simulink model "MSDRPrimaryLoop_LoadFollow"  (R2021b)
settings: Solver=VariableStepAuto  StartTime=0.0  StopTime=604900  MaxStep=1  MinStep=0.01  RelTol=1e-3
undefined symbols (not defined in the file): a_f, A_free_PHX, a_g, A_h_PHX, beta, beta_t, bubbleGeneratorArea, bubbleGeneratorDh, bubbleGeneratorElevation, bubbleGeneratorLength, bubbleGeneratorVolume, bubbleSaturationLevel, bubbleSeparatorArea, bubbleSeparatorDiameter, bubbleSeparatorDo, bubbleSeparatorLength, bubbleSeparatorSlope, bypassRatio, C0, coreFlowArea, coreFuelVolume, coreLowerPlenumArea, coreLowerPlenumHydraulicDiameter, coreLowerPlenumLength, coreLowerPlenumVolume, coreUpperPlenumArea, coreUpperPlenumHydraulicDiameter, coreUpperPlenumLength, coreUpperPlenumVolume, coreVolume, cpGraphite, dissolusionRatio, dMin, dScale, dsmConst, DXeG, Fiss_factor, fuelChannelHydrualicDiameter, fuelChannelLength, fuelDepositRatio, fuelFraction, fuelGraphiteArea, fuelGraphiteHeatTransferCoefficient, gamma0, gamma1, gamma2, generatorDsm, graphiteKDiff, graphiteUnitCellThickness, initialIodineConcentration, InitialXeMolarConcentration, InjectionRatio, injectionRatio, iodineDecayConstant, IodineDecayConstant, iodineYield, kGraphite, kScale, Lam, lam ... (+60)
libraries: fl_lib x268, nesl_utility x106, SimscapeFluids_lib x20, slpidlib x1
(part 1 of 12)
settings Model: PacingRate=4  Creator=silen  LastModifiedBy=silen
settings SolverCC: ZeroCrossAlgorithm=Adaptive
settings DataIOCC: InitialState=xFinal  SaveFinalState=on  SaveOperatingPoint=on  SaveOutput=off  SignalLogging=off  DSMLogging=off  SaveTime=off  ReturnWorkspaceOutputs=off
settings SimscapeCC: SimscapeLogOpenViewer=on

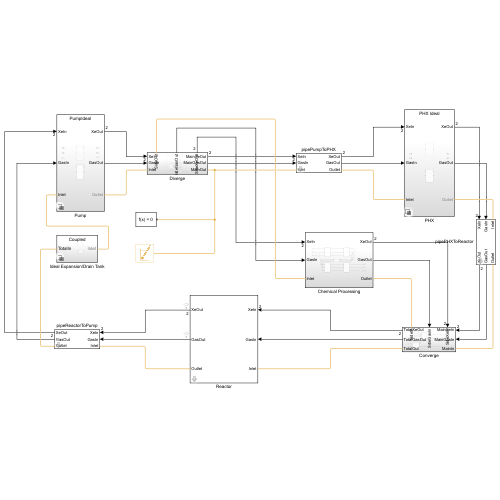
[thumbnail: Simulink's stored preview of the top-level diagram]
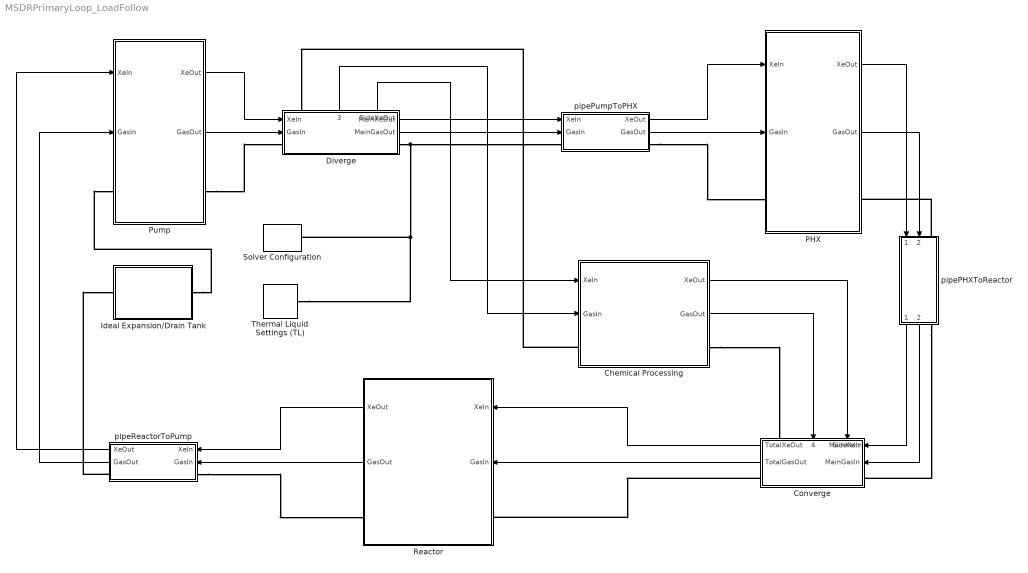
== system MSDRPrimaryLoop_LoadFollow ==
  Chemical Processing : Subsystem
  Converge : Subsystem
      settings: PortSchema="{\"entries\":[{\"content\":{\"sides\":[{\"content\":{\"connectorIds\":[\"In1\",\"In2\",\"LConn1\"]},\"type\":\"ConnectorPlacement.EquallySpacedRectSide\",\"uuid\":\"45a27f6f-7483-4dd0-a911-98512286657b\"},{\"content\":{\"connectorIds\":[\"Out1\",\"Out2\",\"RConn1\"],\"side\":\"RIGHT\"},\"type\":\"ConnectorPlacement.EquallySpacedRectSide\",\"uuid\":\"648a7517-4264-4847-9228-e879d02b25f7\"},{\"content\":{\"connectorIds\":[\"In3\",\"In4\",\"LConn2\"],\"side\":\"TOP\"},\"type\":\"ConnectorPlacement.EquallySpacedRectSide\",\"uuid\":\"a562fb08-ad05-4981-ab1e-7002bfac102c\"},{\"content\":{\"connectorIds\":[],\"side\":\"BOTTOM\"},\"type\":\"ConnectorPlacement.EquallySpacedRectSide\",\"uuid\":\"59ea555a-4c64-4ddd-ae1f-9e1e4b34dfa6\"}]},\"type\":\"ConnectorPlacement.EquallySpacedConnector\",\"uuid\":\"c238e19d-8d7c-41cb-8a15-012ebc62f205\"}],\"packageUris\":[\"http://schema.mathworks.com/mf0/Connector/R2020b\"],\"version\":\"1.0\"}"
  Diverge : Subsystem
      settings: PortSchema="{\"entries\":[{\"content\":{\"sides\":[{\"content\":{\"connectorIds\":[\"In1\",\"In2\",\"LConn1\"]},\"type\":\"ConnectorPlacement.EquallySpacedRectSide\",\"uuid\":\"f25232e3-ff44-4b09-8127-0a17cdec3bda\"},{\"content\":{\"connectorIds\":[\"Out1\",\"Out2\",\"RConn1\"],\"side\":\"RIGHT\"},\"type\":\"ConnectorPlacement.EquallySpacedRectSide\",\"uuid\":\"2b744e7f-4690-47f4-bf66-293fed6e3799\"},{\"content\":{\"connectorIds\":[\"LConn2\",\"Out3\",\"Out4\"],\"side\":\"TOP\"},\"type\":\"ConnectorPlacement.EquallySpacedRectSide\",\"uuid\":\"256231dc-6d03-4995-a517-f1093dd3b2d7\"}]},\"type\":\"ConnectorPlacement.EquallySpacedConnector\",\"uuid\":\"cecb1d8e-0e0f-4899-85a3-e553206939ed\"}],\"packageUris\":[\"http://schema.mathworks.com/mf0/Connector/R2020b\"],\"version\":\"1.0\"}"
  Ideal Expansion/Drain Tank : Subsystem  Variant=on  VariantControlMode=label  VariantControl=Choice  LabelModeActiveChoice=Couple
  PHX : Subsystem  Variant=on  VariantControlMode=label  VariantControl=Choice  LabelModeActiveChoice=Ideal
  Pump : Subsystem  Variant=on  VariantControlMode=label  VariantControl=Choice  LabelModeActiveChoice=Ideal
  Reactor : Subsystem  mask{ReactorPower=thermalPower, NeutronFlux=nominalNeutronFlux}
      mask prompts: ReactorPower "Rated Thermal Power"; NeutronFlux "Nominal Neutron Flux"
  Solver Configuration : nesl_utility/Solver Configuration  PhysicalDomain=network_engine_domain  SubClassName=solver  LeftPortType=input  RightPortType=generic  Tones=[]  Harmonics=[]  SimulateNoise=off  Profile=off  UseLocalSampling=off  EnableSwitchedLinearOptims=on  FrequencyDomain=off  UseCCode=off  RelTol=0.001  AbsTol=1e-06  MinStep=1e-09  ToWorkspace=off  RevertToSquareIcSolve=off  NumHomotopyIterations=100  PhasorMode=off  PhasorModeNumHarmonics=1  DoDC=off  ResidualTolerance=1e-5  UseLocalSolver=on  LocalSolverChoice=NE_BACKWARD_EULER_ADVANCER  LocalSolverSampleTime=1  DoFixedCost=off  MaxNonlinIter=3  MaxModeIter=2  ComputeImpulses=off  ImpulseIterations=2  LinearAlgebra=auto  EquationFormulation=NE_TIME_EF  DelaysMemoryBudget=1024  AutomaticFiltering=on  FilteringTimeConstant=0.001  PartitionStorageMethod=AS_NEEDED  PartitionMemoryBudget=1024  PartitionMethod=ROBUST
      settings: SourceProductBaseCode=PW,SS
  Thermal Liquid Settings (TL) : fl_lib/Thermal Liquid/Utilities/Thermal Liquid Settings (TL)  table_dimensions=foundation.enum.table_dimensions_TL.one_dimensional  T_TLU=temperatureList K  p_TLU=[0.01, 0.1, 5 : 5 : 50] MPa  p_atm=0.1 MPa  pT_region_flag=foundation.enum.pT_region_TL.min_max  T_min=273.16 K  T_max=363.16 K  p_min=0.05 MPa  p_max=50 MPa  T_min_1D=434+273.15 K  T_max_1D=2000+273.15 K  p_min_1D=1 Pa  p_max_1D=10000 MPa  pT_validity_TLU=[1, 1, 1, 1, 1, 1, 1, 1, 1, 1, 1, 1; 1, 1, 1, 1, 1, 1, 1, 1, 1, 1, 1, 1; 1, 1, 1, 1, 1, 1, 1, 1, 1, 1, 1, 1; 1, 1, 1, 1, 1, 1, 1, 1, 1, 1, 1, 1; 1, 1, 1, 1, 1, 1, 1, 1, 1, 1, 1, 1; 0, 1, 1, 1, 1, 1, 1, 1, 1, 1, 1, 1; 0, 1, 1, 1, 1, 1, 1, 1, 1, 1, 1, 1; 0, 1, 1, 1, 1, 1, 1, 1, 1, 1, 1, 1; 0, 1, 1, 1, 1, 1, 1, 1, 1, 1, 1, 1; 0, 1, 1, 1, 1, 1, 1, 1, 1, 1, 1, 1; 0, 0, 1, 1, 1, 1, 1, 1, 1, 1, 1, 1]  rho_parameterization_2D=foundation.enum.rho_parameterization_2D.rho_beta_alpha  rho_parameterization_1D=foundation.enum.rho_parameterization_1D.rho_vector  rho_TLU=[999.7973, 999.8431, 1002.3216, 1004.8218, 1007.293, 1009.7358, 1012.1506, 1014.5379, 1016.8979, 1019.2311, 1021.538, 1023.8188; 999.6579, 999.7009, 1002.0303, 1004.382, 1006.7084, 1009.0101, 1011.2874, 1013.5407, 1015.7703, 1017.9766, 1020.1599, 1022.3206; 998.1632, 998.2045, 1000.4375, 1002.6924, 1004.9239, 1007.1324, 1009.3183, 1011.4819, 1013.6236, 1015.7438, 1017.8428, 1019.921; 995.6057, 995.6458, 997.81864, 1000.0128, 1002.1841, 1004.3332, 1006.4603, 1008.566, 1010.6505, 1012.7144, 1014.758, 1016.7815; 992.1724, 992.2119, 994.35133, 996.5113, 998.6484, 1000.7633, 1002.8563, 1004.928, 1006.9788, 1009.009, 1011.0192, 1013.0097; 988.02, 988.0299, 990.15684, 992.3035, 994.4268, 996.5273, 998.6056, 1000.6622, 1002.6976, 1004.7123, 1006.7067, 1008.6813; 983.18, 983.1901, 985.3217, 987.4721, 989.5983, 991.7008, 993.7803, 995.8374, 997.8726, 999.8864, 1001.8795, 1003.8522; 977.75, 977.7583, 979.9094, 982.0783, 984.2216, 986.34, 988.4343, 990.505, 992.5529, 994.5786, 996.5825, 998.5654; 971.77, 971.7836, 973.96734, 976.1678, 978.3409, 980.4876, 982.6087, 984.7049, 986.7768, 988.8254, 990.8511, 992.8545; 965.26, 965.3023, 967.53107, 969.7753, 971.9901, 974.1764, 976.3354, 978.4676, 980.5741, 982.6556, 984.7129, 986.7465; 958.62, 958.6315, 960.627, 962.9267, 965.1944, 967.4314, 969.6387, 971.8173, 973.9681, 976.0921, 978.19, 980.2628] kg/m^3  beta_TLU=[1.9649, 1.9654, 1.9929, 2.0213, 2.0499, 2.0787, 2.1078, 2.1372, 2.1668, 2.1966, 2.2268, 2.2572; 2.0913, 2.0918, 2.1191, 2.1471, 2.1752, 2.2036, 2.2322, 2.261, 2.2899, 2.3191, 2.3485, 2.3781; 2.1786, 2.1791, 2.2067, 2.235, 2.2634, 2.2919, 2.3206, 2.3494, 2.3784, 2.4075, 2.4367, 2.4661; 2.2332, 2.2337, 2.2619, 2.2908, 2.3197, 2.3487, 2.3778, 2.407, 2.4363, 2.4657, 2.4951, 2.5246; 2.26, 2.2605, 2.2895, 2.3191, 2.3487, 2.3784, 2.4081, 2.4378, 2.4675, 2.4973, 2.5272, 2.5571; 2.2638, 2.2638, 2.2936, 2.324, 2.3544, 2.3848, 2.4151, 2.4455, 2.4758, 2.5062, 2.5365, 2.5669; 2.2472, 2.2472, 2.2779, 2.3092, 2.3403, 2.3715, 2.4025, 2.4336, 2.4646, 2.4955, 2.5264, 2.5573; 2.214, 2.214, 2.2455, 2.2776, 2.3096, 2.3415, 2.3733, 2.405, 2.4367, 2.4683, 2.4998, 2.5313; 2.1668, 2.1668, 2.1992, 2.2321, 2.2649, 2.2976, 2.3301, 2.3626, 2.3949, 2.4272, 2.4593, 2.4914; 2.1081, 2.1081, 2.1413, 2.175, 2.2086, 2.2421, 2.2754, 2.3085, 2.3415, 2.3744, 2.4072, 2.4399; 2.0494, 2.0494, 2.0739, 2.1084, 2.1428, 2.177, 2.211, 2.2449, 2.2786, 2.3121, 2.3455, 2.3788] GPa  alpha_TLU=1e-4 * [-.679, -.676, -.49, -.307, -.13, .041, .206, .365, .519, .668, .811, .949; .878, .881, .998, 1.114, 1.227, 1.337, 1.445, 1.549, 1.651, 1.75, 1.846, 1.939; 2.068, 2.069, 2.141, 2.213, 2.283, 2.352, 2.42, 2.486, 2.551, 2.614, 2.676, 2.736; 3.034, 3.035, 3.074, 3.113, 3.152, 3.191, 3.229, 3.267, 3.305, 3.341, 3.377, 3.413; 3.855, 3.856, 3.87, 3.884, 3.899, 3.914, 3.93, 3.946, 3.961, 3.977, 3.993, 4.009; 4.578, 4.578, 4.572, 4.566, 4.562, 4.558, 4.555, 4.552, 4.55, 4.549, 4.548, 4.547; 5.233, 5.233, 5.209, 5.186, 5.165, 5.144, 5.125, 5.107, 5.09, 5.074, 5.059, 5.045; 5.84, 5.84, 5.801, 5.762, 5.725, 5.691, 5.657, 5.625, 5.595, 5.566, 5.538, 5.512; 6.414, 6.414, 6.36, 6.307, 6.256, 6.208, 6.161, 6.117, 6.074, 6.033, 5.994, 5.956; 6.967, 6.967, 6.898, 6.831, 6.766, 6.705, 6.646, 6.589, 6.535, 6.482, 6.432, 6.384; 7.519, 7.519, 7.423, 7.342, 7.264, 7.189, 7.118, 7.049, 6.983, 6.92, 6.859, 6.8] 1/K  rho_TLU_2=[999.7973, 999.8431, 1002.3216, 1004.8218, 1007.293, 1009.7358, 1012.1506, 1014.5379, 1016.8979, 1019.2311, 1021.538, 1023.8188; 999.6579, 999.7009, 1002.0303, 1004.382, 1006.7084, 1009.0101, 1011.2874, 1013.5407, 1015.7703, 1017.9766, 1020.1599, 1022.3206; 998.1632, 998.2045, 1000.4375, 1002.6924, 1004.9239, 1007.1324, 1009.3183, 1011.4819, 1013.6236, 1015.7438, 1017.8428, 1019.921; 995.6057, 995.6458, 997.81864, 1000.0128, 1002.1841, 1004.3332, 1006.4603, 1008.566, 1010.6505, 1012.7144, 1014.758, 1016.7815; 992.1724, 992.2119, 994.35133, 996.5113, 998.6484, 1000.7633, 1002.8563, 1004.928, 1006.9788, 1009.009, 1011.0192, 1013.0097; 988.02, 988.0299, 990.15684, 992.3035, 994.4268, 996.5273, 998.6056, 1000.6622, 1002.6976, 1004.7123, 1006.7067, 1008.6813; 983.18, 983.1901, 985.3217, 987.4721, 989.5983, 991.7008, 993.7803, 995.8374, 997.8726, 999.8864, 1001.8795, 1003.8522; 977.75, 977.7583, 979.9094, 982.0783, 984.2216, 986.34, 988.4343, 990.505, 992.5529, 994.5786, 996.5825, 998.5654; 971.77, 971.7836, 973.96734, 976.1678, 978.3409, 980.4876, 982.6087, 984.7049, 986.7768, 988.8254, 990.8511, 992.8545; 965.26, 965.3023, 967.53107, 969.7753, 971.9901, 974.1764, 976.3354, 978.4676, 980.5741, 982.6556, 984.7129, 986.7465; 958.62, 958.6315, 960.627, 962.9267, 965.1944, 967.4314, 969.6387, 971.8173, 973.9681, 976.0921, 978.19, 980.2628] kg/m^3  rho_ref_3=998.21 kg/m^3  T_ref_3=293.16 K  p_ref_3=0.101325 MPa  beta_const_3=2.1791 GPa  alpha_const_3=2.0691e-4 1/K  rho_TLU_4=rhoList kg/m^3  beta_const_4=20 GPa  p_ref_4=0.101325 MPa  rho_ref_5=998.21 kg/m^3  T_ref_5=293.16 K  p_ref_5=0.101325 MPa  beta_const_5=2.1791 GPa  alpha_const_5=2.0691e-4 1/K  u_parameterization_2D=foundation.enum.u_parameterization_2D.u_cp  u_parameterization_1D=foundation.enum.u_parameterization_1D.cp  u_TLU=[.0002, .0018, .086, .1588, .219, .267, .3034, .3288, .3436, .3483, .3435, .3294; 42.062, 42.06, 41.935, 41.804, 41.668, 41.527, 41.382, 41.233, 41.081, 40.924, 40.763, 40.599; 83.953, 83.948, 83.651, 83.349, 83.049, 82.749, 82.451, 82.153, 81.856, 81.56, 81.265, 80.971; 125.77, 125.76, 125.31, 124.86, 124.41, 123.97, 123.53, 123.1, 122.68, 122.25, 121.84, 121.42; 167.57, 167.56, 166.96, 166.37, 165.79, 165.21, 164.65, 164.09, 163.54, 163, 162.46, 161.94; 209.36, 209.36, 208.63, 207.9, 207.19, 206.48, 205.79, 205.11, 204.45, 203.79, 203.14, 202.5; 251.19, 251.19, 250.33, 249.47, 248.62, 247.79, 246.98, 246.18, 245.39, 244.62, 243.86, 243.12; 293.06, 293.06, 292.07, 291.07, 290.1, 289.14, 288.2, 287.28, 286.38, 285.49, 284.62, 283.77; 334.99, 334.99, 333.86, 332.73, 331.63, 330.54, 329.48, 328.44, 327.41, 326.41, 325.43, 324.46; 377, 377, 375.73, 374.46, 373.22, 372, 370.81, 369.64, 368.5, 367.38, 366.27, 365.19; 419.01, 419.01, 417.69, 416.27, 414.89, 413.54, 412.21, 410.91, 409.64, 408.4, 407.17, 405.98] kJ/kg  cp_TLU=[4.2199, 4.2194, 4.1957, 4.1726, 4.1508, 4.13, 4.1103, 4.0916, 4.0738, 4.0569, 4.0408, 4.0254; 4.1955, 4.1951, 4.1769, 4.1592, 4.1422, 4.1259, 4.1103, 4.0954, 4.0812, 4.0676, 4.0545, 4.0421; 4.1843, 4.184, 4.169, 4.1543, 4.1401, 4.1264, 4.1133, 4.1007, 4.0885, 4.0768, 4.0656, 4.0548; 4.1801, 4.1798, 4.1667, 4.1538, 4.1413, 4.1293, 4.1177, 4.1064, 4.0956, 4.0851, 4.075, 4.0653; 4.1796, 4.1794, 4.1675, 4.1558, 4.1444, 4.1334, 4.1227, 4.1123, 4.1023, 4.0926, 4.0832, 4.0741; 4.1813, 4.1813, 4.1702, 4.1592, 4.1484, 4.138, 4.1279, 4.1181, 4.1086, 4.0993, 4.0903, 4.0816; 4.185, 4.185, 4.1742, 4.1636, 4.1532, 4.1432, 4.1334, 4.1239, 4.1146, 4.1056, 4.0969, 4.0884; 4.1901, 4.1901, 4.1795, 4.169, 4.1588, 4.1489, 4.1393, 4.1299, 4.1207, 4.1118, 4.1032, 4.0947; 4.1968, 4.1968, 4.1862, 4.1757, 4.1655, 4.1555, 4.1458, 4.1364, 4.1273, 4.1183, 4.1096, 4.1012; 4.2052, 4.2052, 4.1944, 4.1837, 4.1733, 4.1632, 4.1534, 4.1438, 4.1345, 4.1255, 4.1166, 4.108; 4.2136, 4.2136, 4.2045, 4.1935, 4.1828, 4.1724, 4.1623, 4.1524, 4.1429, 4.1335, 4.1245, 4.1157] kJ/(K*kg)  u_TLU_2=[.0002, .0018, .086, .1588, .219, .267, .3034, .3288, .3436, .3483, .3435, .3294; 42.062, 42.06, 41.935, 41.804, 41.668, 41.527, 41.382, 41.233, 41.081, 40.924, 40.763, 40.599; 83.953, 83.948, 83.651, 83.349, 83.049, 82.749, 82.451, 82.153, 81.856, 81.56, 81.265, 80.971; 125.77, 125.76, 125.31, 124.86, 124.41, 123.97, 123.53, 123.1, 122.68, 122.25, 121.84, 121.42; 167.57, 167.56, 166.96, 166.37, 165.79, 165.21, 164.65, 164.09, 163.54, 163, 162.46, 161.94; 209.36, 209.36, 208.63, 207.9, 207.19, 206.48, 205.79, 205.11, 204.45, 203.79, 203.14, 202.5; 251.19, 251.19, 250.33, 249.47, 248.62, 247.79, 246.98, 246.18, 245.39, 244.62, 243.86, 243.12; 293.06, 293.06, 292.07, 291.07, 290.1, 289.14, 288.2, 287.28, 286.38, 285.49, 284.62, 283.77; 334.99, 334.99, 333.86, 332.73, 331.63, 330.54, 329.48, 328.44, 327.41, 326.41, 325.43, 324.46; 377, 377, 375.73, 374.46, 373.22, 372, 370.81, 369.64, 368.5, 367.38, 366.27, 365.19; 419.01, 419.01, 417.69, 416.27, 414.89, 413.54, 412.21, 410.91, 409.64, 408.4, 407.17, 405.98] kJ/kg  cp_TLU_3=[4.2199, 4.2194, 4.1957, 4.1726, 4.1508, 4.13, 4.1103, 4.0916, 4.0738, 4.0569, 4.0408, 4.0254; 4.1955, 4.1951, 4.1769, 4.1592, 4.1422, 4.1259, 4.1103, 4.0954, 4.0812, 4.0676, 4.0545, 4.0421; 4.1843, 4.184, 4.169, 4.1543, 4.1401, 4.1264, 4.1133, 4.1007, 4.0885, 4.0768, 4.0656, 4.0548; 4.1801, 4.1798, 4.1667, 4.1538, 4.1413, 4.1293, 4.1177, 4.1064, 4.0956, 4.0851, 4.075, 4.0653; 4.1796, 4.1794, 4.1675, 4.1558, 4.1444, 4.1334, 4.1227, 4.1123, 4.1023, 4.0926, 4.0832, 4.0741; 4.1813, 4.1813, 4.1702, 4.1592, 4.1484, 4.138, 4.1279, 4.1181, 4.1086, 4.0993, 4.0903, 4.0816; 4.185, 4.185, 4.1742, 4.1636, 4.1532, 4.1432, 4.1334, 4.1239, 4.1146, 4.1056, 4.0969, 4.0884; 4.1901, 4.1901, 4.1795, 4.169, 4.1588, 4.1489, 4.1393, 4.1299, 4.1207, 4.1118, 4.1032, 4.0947; 4.1968, 4.1968, 4.1862, 4.1757, 4.1655, 4.1555, 4.1458, 4.1364, 4.1273, 4.1183, 4.1096, 4.1012; 4.2052, 4.2052, 4.1944, 4.1837, 4.1733, 4.1632, 4.1534, 4.1438, 4.1345, 4.1255, 4.1166, 4.108; 4.2136, 4.2136, 4.2045, 4.1935, 4.1828, 4.1724, 4.1623, 4.1524, 4.1429, 4.1335, 4.1245, 4.1157] kJ/(K*kg)  u_TLU_4=[.0018; 42.06; 83.948; 125.76; 167.56; 209.36; 251.19; 293.06; 334.99; 377; 418.01] kJ/kg  cp_TLU_5=cpList J/(K*kg)  nu_TLU=[1.7917, 1.7914, 1.7763, 1.7615, 1.7473, 1.7338, 1.7208, 1.7085, 1.6967, 1.6854, 1.6747, 1.6645; 1.3061, 1.3059, 1.2986, 1.2914, 1.2845, 1.2779, 1.2716, 1.2656, 1.2598, 1.2543, 1.2491, 1.2441; 1.0032, 1.0032, .9995, .9959, .9924, .9891, .9859, .9829, .9801, .9774, .9748, .9724; .8006, .8005, .7987, .797, .7953, .7937, .7922, .7908, .7894, .7881, .787, .7859; .6577, .6577, .657, .6562, .6555, .6548, .6543, .6537, .6532, .6528, .6523, .652; .553, .553, .5529, .5527, .5526, .5525, .5524, .5524, .5524, .5524, .5524, .5525; .4739, .4739, .4741, .4743, .4745, .4747, .475, .4753, .4755, .4758, .4762, .4765; .4127, .4127, .4131, .4135, .4139, .4143, .4148, .4152, .4157, .4162, .4167, .4172; .3643, .3643, .3648, .3654, .3659, .3665, .367, .3676, .3682, .3688, .3694, .37; .3254, .3254, .3261, .3267, .3273, .328, .3286, .3293, .3299, .3306, .3312, .3319; .2866, .2866, .2945, .2952, .2959, .2965, .2972, .2979, .2986, .2993, .3, .3007] mm^2/s  nu_TLU_2=nuList m^2/s  k_TLU=[561.04, 561.09, 563.8, 566.56, 569.32, 572.08, 574.82, 577.54, 580.24, 582.92, 585.57, 588.18; 580.02, 580.07, 582.45, 584.88, 587.32, 589.75, 592.18, 594.61, 597.02, 599.42, 601.8, 604.16; 598.44, 598.48, 600.73, 603.03, 605.33, 607.64, 609.94, 612.24, 614.54, 616.82, 619.1, 621.36; 615.48, 615.52, 617.73, 620, 622.26, 624.54, 626.81, 629.07, 631.34, 633.6, 635.85, 638.09; 630.6, 630.64, 632.87, 635.15, 637.44, 639.72, 642.01, 644.29, 646.57, 648.84, 651.11, 653.36; 643.61, 643.61, 645.88, 648.21, 650.53, 652.86, 655.18, 657.51, 659.82, 662.14, 664.44, 666.74; 654.39, 654.39, 656.73, 659.12, 661.5, 663.89, 666.27, 668.65, 671.02, 673.38, 675.74, 678.09; 663.13, 663.13, 665.54, 668, 670.46, 672.91, 675.36, 677.8, 680.24, 682.67, 685.09, 687.5; 670.02, 670.02, 672.51, 675.05, 677.59, 680.12, 682.64, 685.16, 687.67, 690.17, 692.66, 695.14; 675.27, 675.27, 677.85, 680.48, 683.11, 685.73, 688.34, 690.94, 693.53, 696.11, 698.68, 701.24; 680.52, 680.52, 681.77, 684.5, 687.22, 689.94, 692.64, 695.34, 698.02, 700.69, 703.35, 706] mW/(K*m)  k_TLU_2=conductivityList W/(m*K)
      settings: SourceProductBaseCode=SS
  pipePHXToReactor : Subsystem  mask{Volume=pipePHXToReactorVolume, Area=pipeArea, Length=pipePHXToReactorLength, Dh=pipeID, Elevation=pipePHXToReactorElevation}
      mask prompts: Dh "Hydraulic Diameter"
  pipePumpToPHX : Subsystem  mask{Volume=pipePumpToPHXVolume, Area=pipeArea, Length=pipePumpToPHXLength, Dh=pipeID, Elevation=pipePumpToPHXElevation}
      mask prompts: Dh "Hydraulic Diameter"
  pipeReactorToPump : Subsystem  mask{Volume=pipeReactorToPumpVolume, Area=pipeArea, Length=pipeReactorToPumpLength, Dh=pipeID, Elevation=pipeReactorToPumpElevation}
      mask prompts: Dh "Hydraulic Diameter"
  wires:
  pipeReactorToPump/2(GasOut) -> Pump/2(GasIn)
  Reactor/2(GasOut) -> pipeReactorToPump/2(GasIn)
  pipeReactorToPump/1(XeOut) -> Pump/1(XeIn)
  Reactor/1(XeOut) -> pipeReactorToPump/1(XeIn)
  Diverge/4(SideXeOut) -> Chemical Processing/1(XeIn)
  Diverge/3(SideGasOut) -> Chemical Processing/2(GasIn)
  Chemical Processing/2(GasOut) -> Converge/4(SdieGasIn)
  Chemical Processing/1(XeOut) -> Converge/3(SideXeIn)
  Diverge/2(MainGasOut) -> pipePumpToPHX/2(GasIn)
  Diverge/1(MainXeOut) -> pipePumpToPHX/1(XeIn)
  Pump/1(XeOut) -> Diverge/1(XeIn)
  Pump/2(GasOut) -> Diverge/2(GasIn)
  pipePumpToPHX/2(GasOut) -> PHX/2(GasIn)
  pipePumpToPHX/1(XeOut) -> PHX/1(XeIn)
  pipePHXToReactor/1(XeOut) -> Converge/1(MainXeIn)
  pipePHXToReactor/2(GasOut) -> Converge/2(MainGasIn)
  Converge/2(TotalGasOut) -> Reactor/2(GasIn)
  Converge/1(TotalXeOut) -> Reactor/1(XeIn)
  PHX/2(GasOut) -> pipePHXToReactor/2(GasIn)
  PHX/1(XeOut) -> pipePHXToReactor/1(XeIn)
  connections:
  Chemical Processing/RConn1 -- Converge/LConn2
  Chemical Processing/LConn1 -- Diverge/LConn2
  pipeReactorToPump/RConn1 -- Ideal Expansion/Drain Tank/LConn1
  Ideal Expansion/Drain Tank/RConn1 -- Pump/LConn1
  Diverge/RConn1 -- Thermal Liquid Settings (TL)/RConn1 -- Solver Configuration/RConn1 -- pipePumpToPHX/LConn1
  Pump/RConn1 -- Diverge/LConn1
  pipePumpToPHX/RConn1 -- PHX/LConn1
  pipePHXToReactor/RConn1 -- Converge/LConn1
  Converge/RConn1 -- Reactor/LConn1
  pipePHXToReactor/LConn1 -- PHX/RConn1
  pipeReactorToPump/LConn1 -- Reactor/RConn1

== system MSDRPrimaryLoop_LoadFollow/Chemical Processing ==
  XeIn : Inport
  GasIn : Inport  Port=2
  Bubble Generator : Subsystem
  Bubble Separator : Subsystem
  ElevationPipe : Subsystem  mask{Volume=pipeLineArea*pipePHXToReactorLength, Area=pipeLineArea, Length=pipePHXToReactorLength, Dh=pipeLineDh, Elevation=pipePHXToReactorElevation}
      mask prompts: Dh "Hydraulic Diameter"
  PipeLine : Subsystem
  VariablePressureControl : Subsystem
  Inlet : PMIOPort  Side=Left
  Outlet : PMIOPort  Port=2  Side=Right
  XeOut : Outport
  GasOut : Outport  Port=2
  wires:
  XeIn/1 -> Bubble Generator/1(XeIn)
  GasIn/1 -> Bubble Generator/2(GasIn)
  Bubble Generator/2(GasOut) -> PipeLine/2(GasIn)
  Bubble Generator/1(XeOut) -> PipeLine/1(XeIn)
  Bubble Separator/1(XeOut) -> VariablePressureControl/1(XeIn)
  Bubble Separator/2(GasOut) -> VariablePressureControl/2(GasIn)
  VariablePressureControl/2(GasOut) -> GasOut/1
  VariablePressureControl/1(XeOut) -> XeOut/1
  PipeLine/2(GasOut) -> ElevationPipe/2(GasIn)
  ElevationPipe/2(GasOut) -> Bubble Separator/2(GasIn)
  PipeLine/1(XeOut) -> ElevationPipe/1(XeIn)
  ElevationPipe/1(XeOut) -> Bubble Separator/1(XeIn)
  connections:
  PipeLine/LConn1 -- Bubble Generator/RConn1
  VariablePressureControl/LConn1 -- Bubble Separator/RConn1
  PipeLine/RConn1 -- ElevationPipe/LConn1
  ElevationPipe/RConn1 -- Bubble Separator/LConn1
  Outlet/RConn1 -- VariablePressureControl/RConn1
  Bubble Generator/LConn1 -- Inlet/RConn1

== system MSDRPrimaryLoop_LoadFollow/Converge ==
  MainXeIn : Inport
  MainGasIn : Inport  Port=2
  SideXeIn : Inport  Port=3
  SdieGasIn : Inport  Port=4
  Mixing : Subsystem
  PhysicalNetwork : Subsystem
  MainIn : PMIOPort  Side=Left
  SideIn : PMIOPort  Port=2  Side=Left
  TotalOut : PMIOPort  Port=3  Side=Right
  TotalXeOut : Outport
  TotalGasOut : Outport  Port=2
  wires:
  Mixing/2(GasOut) -> TotalGasOut/1
  Mixing/1(XeOut) -> TotalXeOut/1
  SdieGasIn/1 -> Mixing/4(Gas2)
  MainGasIn/1 -> Mixing/3(Gas1)
  MainXeIn/1 -> Mixing/1(Xe1)
  SideXeIn/1 -> Mixing/2(Xe2)
  connections:
  PhysicalNetwork/RConn3 -- TotalOut/RConn1
  PhysicalNetwork/RConn1 -- Mixing/LConn1
  PhysicalNetwork/RConn2 -- Mixing/LConn2
  PhysicalNetwork/LConn1 -- MainIn/RConn1
  PhysicalNetwork/LConn2 -- SideIn/RConn1

== system MSDRPrimaryLoop_LoadFollow/Diverge ==
  XeIn : Inport
  GasIn : Inport  Port=2
  GasExpansion : Subsystem  ReferencedSubsystem=GasExpansion
      settings: PortSchema="{\"entries\":[{\"content\":{\"sides\":[{\"content\":{\"connectorIds\":[\"LConn1\",\"In1\"]},\"type\":\"ConnectorPlacement.EquallySpacedRectSide\",\"uuid\":\"50c89675-cb8a-4964-af62-cb2014507b1d\"},{\"content\":{\"connectorIds\":[\"RConn1\",\"Out1\"],\"side\":\"RIGHT\"},\"type\":\"ConnectorPlacement.EquallySpacedRectSide\",\"uuid\":\"6b3adc78-0be5-4682-9da0-6fd41ffc4e71\"},{\"content\":{\"connectorIds\":[],\"side\":\"TOP\"},\"type\":\"ConnectorPlacement.EquallySpacedRectSide\",\"uuid\":\"5158b46f-a496-48e4-90d6-6c6dcc9e237b\"}]},\"type\":\"ConnectorPlacement.EquallySpacedConnector\",\"uuid\":\"7ff0188e-dc19-44a0-a8cf-bde33949414f\"}],\"packageUris\":[\"http://schema.mathworks.com/mf0/Connector/R2020b\"],\"version\":\"1.0\"}"
  GasExpansion1 : Subsystem  ReferencedSubsystem=GasExpansion
      settings: PortSchema="{\"entries\":[{\"content\":{\"sides\":[{\"content\":{\"connectorIds\":[\"LConn1\",\"In1\"]},\"type\":\"ConnectorPlacement.EquallySpacedRectSide\",\"uuid\":\"50c89675-cb8a-4964-af62-cb2014507b1d\"},{\"content\":{\"connectorIds\":[\"RConn1\",\"Out1\"],\"side\":\"RIGHT\"},\"type\":\"ConnectorPlacement.EquallySpacedRectSide\",\"uuid\":\"6b3adc78-0be5-4682-9da0-6fd41ffc4e71\"},{\"content\":{\"connectorIds\":[],\"side\":\"TOP\"},\"type\":\"ConnectorPlacement.EquallySpacedRectSide\",\"uuid\":\"5158b46f-a496-48e4-90d6-6c6dcc9e237b\"}]},\"type\":\"ConnectorPlacement.EquallySpacedConnector\",\"uuid\":\"7ff0188e-dc19-44a0-a8cf-bde33949414f\"}],\"packageUris\":[\"http://schema.mathworks.com/mf0/Connector/R2020b\"],\"version\":\"1.0\"}"
  Product : Product
  Product1 : Product
  Subsystem1 : Subsystem
  Inlet : PMIOPort  Side=Left
  SideOut : PMIOPort  Port=2  Side=Left
  MainOut : PMIOPort  Port=3  Side=Right
  MainXeOut : Outport
  MainGasOut : Outport  Port=2
  SideGasOut : Outport  Port=3
  SideXeOut : Outport  Port=4
  wires:
  Subsystem1/2(SideRatio) -> Product1/2
  XeIn/1 -> Product1/1, Product/1
  GasIn/1 -> GasExpansion1/1, GasExpansion/1
  Product1/1 -> SideXeOut/1
  Subsystem1/1(MainRatio) -> Product/2
  Product/1 -> MainXeOut/1
  GasExpansion/1 -> MainGasOut/1
  GasExpansion1/1 -> SideGasOut/1
  connections:
  Subsystem1/LConn1 -- Inlet/RConn1 -- GasExpansion1/LConn1 -- GasExpansion/LConn1
  Subsystem1/RConn1 -- GasExpansion/RConn1 -- MainOut/RConn1
  Subsystem1/RConn2 -- GasExpansion1/RConn1 -- SideOut/RConn1

== system MSDRPrimaryLoop_LoadFollow/Ideal Expansion//Drain Tank ==
  Coupled : Subsystem  VariantControl=Couple
  Segregate : Subsystem  VariantControl=Segregate
  TotalIn : PMIOPort  Side=Left
  Inlet : PMIOPort  Port=2  Side=Right

== system MSDRPrimaryLoop_LoadFollow/PHX ==
  XeIn : Inport
  GasIn : Inport  Port=2
  PHX Ideal : Subsystem  VariantControl=Ideal  mask{PHXVolume=PHXFuelVolume*2, FlowArea=PHXFuelVolume/PHXLength*2, TOut=nominalPHXSaltOutTemp, dP=nominalPHXPressureLoss, VDot=nominalDischargeRate*0.9}
      mask prompts: PHXVolume "Fuel Volume Inventory"; FlowArea "Total Flow Area"; TOut "Design Outlet Temperature"; dP "Deisgn Pressure Loss"; VDot "Design Flow Rate"
  PHX Physical : Subsystem  VariantControl=Physical  mask{PHXVolume=PHXVolume, FlowArea=A_free_PHX, ChannelLength=PHXVolume/A_free_PHX, Dh=0.0254*0.305, HeatExchangeArea=A_h_PHX}
      mask prompts: PHXVolume "Fuel Volume Inventory"; FlowArea "Total Flow Area"; ChannelLength "Channel Length"; Dh "Tube Hydraulic Diameter"; HeatExchangeArea "Heat Exchange Area"
  Inlet : PMIOPort  Side=Left
  Outlet : PMIOPort  Port=2  Side=Right
  XeOut : Outport
  GasOut : Outport  Port=2

== system MSDRPrimaryLoop_LoadFollow/Pump ==
  XeIn : Inport
  GasIn : Inport  Port=2
  PumpIdeal : Subsystem  VariantControl=Ideal  mask{PumpVolume=pumpVolume, VDot=nominalDischargeRate}
      mask prompts: PumpVolume "Pump Volume"; VDot "Design Flow Rate"
  PumpPysical : Subsystem  VariantControl=Physical
  Inlet : PMIOPort  Side=Left
  Outlet : PMIOPort  Port=2  Side=Right
  XeOut : Outport
  GasOut : Outport  Port=2

== system MSDRPrimaryLoop_LoadFollow/Reactor ==
  XeIn : Inport
  GasIn : Inport  Port=2
  CoreTH&Inerti : Subsystem  mask{CoreVolume=coreVolume, CoreFlowArea=coreFlowArea, CoreLength=fuelChannelLength, FuelFraction=fuelFraction, Dh=fuelChannelHydrualicDiameter, UPVolume=coreUpperPlenumVolume, LPVolume=coreLowerPlenumVolume, FuelGraphiteArea=fuelGraphiteArea, FuelInCoreRatio=coreFuelVolume/(coreFuelVolume+outCoreFuelVolume)}
      mask prompts: CoreVolume "Core Volume"; CoreFlowArea "Flow Area"; CoreLength "Flow Channel Length"; FuelFraction "Fuel Fraction"; Dh "Unit Cell Hydraulic Diameter"; UPVolume "Upper Plenum Volume"; LPVolume "Lower Plenum Volume"; FuelGraphiteArea "Fuel-Graphite Interface Area"; FuelInCoreRatio "Fuel In Core Ratio"
      settings: PortSchema="{\"entries\":[{\"content\":{\"sides\":[{\"content\":{\"connectorIds\":[\"In1\",\"In2\",\"LConn1\"]},\"type\":\"ConnectorPlacement.EquallySpacedRectSide\",\"uuid\":\"ded74b10-d98f-4cd8-855f-58264db5fd15\"},{\"content\":{\"connectorIds\":[\"Out1\",\"Out2\",\"RConn1\"],\"side\":\"RIGHT\"},\"type\":\"ConnectorPlacement.EquallySpacedRectSide\",\"uuid\":\"0585ebfb-4248-46bd-bca6-54c57d7b6442\"},{\"content\":{\"connectorIds\":[\"Out4\"],\"side\":\"TOP\"},\"type\":\"ConnectorPlacement.EquallySpacedRectSide\",\"uuid\":\"9174621e-d574-4f3d-89f3-8bac9d6be5e6\"},{\"content\":{\"connectorIds\":[\"In3\",\"In4\",\"In5\",\"Out3\"],\"side\":\"BOTTOM\"},\"type\":\"ConnectorPlacement.EquallySpacedRectSide\",\"uuid\":\"122afcef-c2c4-4310-aa73-fffd11424b5e\"}]},\"type\":\"ConnectorPlacement.EquallySpacedConnector\",\"uuid\":\"036fff48-b906-409b-bf0b-28cd7e945db0\"}],\"packageUris\":[\"http://schema.mathworks.com/mf0/Connector/R2020b\"],\"version\":\"1.0\"}"
  Decay Heat : Subsystem
  Delay One Step : Delay  DelayLength=1  InitialCondition=1
  Delay One Step1 : Delay  DelayLength=1  InitialCondition=0
  Delay One Step2 : Delay  DelayLength=1  InitialCondition=0
  FlowFraction : Subsystem
      settings: PortSchema="{\"entries\":[{\"content\":{\"sides\":[{\"content\":{\"connectorIds\":[\"LConn1\"]},\"type\":\"ConnectorPlacement.EquallySpacedRectSide\",\"uuid\":\"00cace53-f293-4248-b217-dcf15c2e9f69\"},{\"content\":{\"connectorIds\":[\"RConn1\"],\"side\":\"RIGHT\"},\"type\":\"ConnectorPlacement.EquallySpacedRectSide\",\"uuid\":\"216c6044-34ad-4385-b65d-f279c2ecb83d\"},{\"content\":{\"connectorIds\":[],\"side\":\"TOP\"},\"type\":\"ConnectorPlacement.EquallySpacedRectSide\",\"uuid\":\"46130bf8-f250-4038-a587-23e05e5fbaf6\"},{\"content\":{\"connectorIds\":[\"Out1\"],\"side\":\"BOTTOM\"},\"type\":\"ConnectorPlacement.EquallySpacedRectSide\",\"uuid\":\"e6da8c2a-dbf4-4d10-8882-686f425d2699\"}]},\"type\":\"ConnectorPlacement.EquallySpacedConnector\",\"uuid\":\"8f661642-16f9-490f-b3f8-cd6ea725baf7\"}],\"packageUris\":[\"http://schema.mathworks.com/mf0/Connector/R2020b\"],\"version\":\"1.0\"}"
  Iodine : Subsystem  mask{TotalFuelMass=(coreFuelVolume+3*outCoreFuelVolume)*nominalFuelDensity}
      mask prompts: TotalFuelMass "Total Fuel Mass"
  Reactivity&PKE : Subsystem  Variant=on  VariantControlMode=label  VariantControl=Choice  LabelModeActiveChoice=Ideal
      settings: PortSchema="{\"entries\":[{\"content\":{\"sides\":[{\"content\":{\"connectorIds\":[]},\"type\":\"ConnectorPlacement.EquallySpacedRectSide\",\"uuid\":\"9a7ecffa-f301-4611-a629-37819faea5ef\"},{\"content\":{\"connectorIds\":[\"In2\",\"In3\"],\"side\":\"RIGHT\"},\"type\":\"ConnectorPlacement.EquallySpacedRectSide\",\"uuid\":\"cf44784b-28b7-4f05-b998-f6795a1cd2c6\"},{\"content\":{\"connectorIds\":[\"In1\"],\"side\":\"TOP\"},\"type\":\"ConnectorPlacement.EquallySpacedRectSide\",\"uuid\":\"595678e9-b0c5-4855-b1a3-7610b2b455b4\"},{\"content\":{\"connectorIds\":[\"Out1\"],\"side\":\"BOTTOM\"},\"type\":\"ConnectorPlacement.EquallySpacedRectSide\",\"uuid\":\"49c56d9c-c7fe-43b5-bc79-4a2499eb532c\"}]},\"type\":\"ConnectorPlacement.EquallySpacedConnector\",\"uuid\":\"68419379-3a11-4cd2-b73f-bd3b6a83d121\"}],\"packageUris\":[\"http://schema.mathworks.com/mf0/Connector/R2020b\"],\"version\":\"1.0\"}"
  Inlet : PMIOPort  Side=Left
  Outlet : PMIOPort  Port=2  Side=Right
  XeOut : Outport
  GasOut : Outport  Port=2
  tag scope: IodineSNDensity=global
  wires:
  XeIn/1 -> CoreTH&Inerti/1(XeIn)
  GasIn/1 -> CoreTH&Inerti/2(GasIn)
  CoreTH&Inerti/1(XeOut) -> XeOut/1
  CoreTH&Inerti/2(GasOut) -> GasOut/1
  Decay Heat/1("Relative Decay Power ") -> Delay One Step2/1
  Iodine/1(IodineSpecificNumberDensity) -> Delay One Step1/1
  FlowFraction/1(FlowFrac) -> Reactivity&PKE/2(FlowFrac)
  Delay One Step/1 -> CoreTH&Inerti/5(NeutronFraction)
  Delay One Step1/1 -> [IodineSNDensity], CoreTH&Inerti/4(IodineNumberDensity)
  Delay One Step2/1 -> CoreTH&Inerti/3(DecayFraction)
  CoreTH&Inerti/4("XeCore, [cm^2]") -> Reactivity&PKE/1("XeCore, [cm^2]")
  CoreTH&Inerti/3(Temperatures) -> Reactivity&PKE/3(CORE TEMPERATURE)
  Reactivity&PKE/1(FRACTIONAL NEUTRON DENSITY) -> Delay One Step/1, Iodine/1(NeutronFraction), Decay Heat/1((n/n_0))
  connections:
  FlowFraction/LConn1 -- Outlet/RConn1
  CoreTH&Inerti/RConn1 -- FlowFraction/RConn1
  Inlet/RConn1 -- CoreTH&Inerti/LConn1

== system MSDRPrimaryLoop_LoadFollow/pipePHXToReactor ==
  XeIn : Inport
  GasIn : Inport  Port=2
  Add : Sum  Inputs=|++
  Delay One Step : Delay  DelayLength=1
  Gain : Gain  Gain=0.5
  GasCalc : Subsystem  mask{Volume=Volume}
      settings: PortSchema="{\"entries\":[{\"content\":{\"sides\":[{\"content\":{\"connectorIds\":[\"In1\"]},\"type\":\"ConnectorPlacement.EquallySpacedRectSide\",\"uuid\":\"a8e1ce06-71c9-462d-8d5c-7a3e078b5544\"},{\"content\":{\"connectorIds\":[\"Out1\"],\"side\":\"RIGHT\"},\"type\":\"ConnectorPlacement.EquallySpacedRectSide\",\"uuid\":\"2c63a1ce-15e2-4b17-a432-f9f40781bd58\"},{\"content\":{\"connectorIds\":[\"LConn1\",\"LConn2\",\"LConn3\"],\"side\":\"TOP\"},\"type\":\"ConnectorPlacement.EquallySpacedRectSide\",\"uuid\":\"abc20e07-15eb-475f-be7f-cc96378523a1\"},{\"content\":{\"connectorIds\":[],\"side\":\"BOTTOM\"},\"type\":\"ConnectorPlacement.EquallySpacedRectSide\",\"uuid\":\"ab58f362-f4c2-4e86-bda0-802426066295\"}]},\"type\":\"ConnectorPlacement.EquallySpacedConnector\",\"uuid\":\"b54d49a9-048b-4912-bf18-92a7ef5e8aff\"}],\"packageUris\":[\"http://schema.mathworks.com/mf0/Connector/R2020b\"],\"version\":\"1.0\"}"
  PLossFunc : Subsystem
      settings: PortSchema="{\"entries\":[{\"content\":{\"sides\":[{\"content\":{\"connectorIds\":[\"Out1\",\"LConn1\"]},\"type\":\"ConnectorPlacement.EquallySpacedRectSide\",\"uuid\":\"95ca4545-c473-4e31-844b-c43557042c16\"},{\"content\":{\"connectorIds\":[\"RConn1\"],\"side\":\"RIGHT\"},\"type\":\"ConnectorPlacement.EquallySpacedRectSide\",\"uuid\":\"f9304c30-8684-4a05-a34b-3121610e628d\"},{\"content\":{\"connectorIds\":[],\"side\":\"TOP\"},\"type\":\"ConnectorPlacement.EquallySpacedRectSide\",\"uuid\":\"64c7a4d8-8539-4303-ae81-4015bd1451af\"}]},\"type\":\"ConnectorPlacement.EquallySpacedConnector\",\"uuid\":\"40c12b2f-fb9d-4a19-b6f1-e93ae1fd4d68\"}],\"packageUris\":[\"http://schema.mathworks.com/mf0/Connector/R2020b\"],\"version\":\"1.0\"}"
  Subsystem : Subsystem  mask{Volume=Volume, Area=Area, Length=Length, Dh=Dh, Elevation=Elevation}
      mask prompts: Dh "Hydraulic Diameter"
      settings: PortSchema="{\"entries\":[{\"content\":{\"sides\":[{\"content\":{\"connectorIds\":[\"LConn1\",\"In1\"]},\"type\":\"ConnectorPlacement.EquallySpacedRectSide\",\"uuid\":\"0f255306-ec83-4423-ac41-a2708bd1ec44\"},{\"content\":{\"connectorIds\":[\"RConn1\"],\"side\":\"RIGHT\"},\"type\":\"ConnectorPlacement.EquallySpacedRectSide\",\"uuid\":\"650fb4ea-7b32-4c45-8538-9785d9ca64bf\"},{\"content\":{\"connectorIds\":[],\"side\":\"TOP\"},\"type\":\"ConnectorPlacement.EquallySpacedRectSide\",\"uuid\":\"434d3568-54a4-4787-a287-69f15ef478cb\"},{\"content\":{\"connectorIds\":[\"RConn2\"],\"side\":\"BOTTOM\"},\"type\":\"ConnectorPlacement.EquallySpacedRectSide\",\"uuid\":\"5b0b510d-1175-4508-bbe9-65b563e28484\"}]},\"type\":\"ConnectorPlacement.EquallySpacedConnector\",\"uuid\":\"b18d9c84-3d71-444b-a89d-79c3dc70d4d9\"}],\"packageUris\":[\"http://schema.mathworks.com/mf0/Connector/R2020b\"],\"version\":\"1.0\"}"
  XenonCalc : Subsystem  mask{Volume=Volume, Area=Area, Length=Length, Dh=Dh, Elevation=Elevation}
      mask prompts: Dh "Hydraulic Diameter"
      settings: PortSchema="{\"entries\":[{\"content\":{\"sides\":[{\"content\":{\"connectorIds\":[\"LConn1\",\"In1\"]},\"type\":\"ConnectorPlacement.EquallySpacedRectSide\",\"uuid\":\"82f8e7e7-fd89-4597-952e-64db268d0190\"},{\"content\":{\"connectorIds\":[\"RConn1\",\"Out1\"],\"side\":\"RIGHT\"},\"type\":\"ConnectorPlacement.EquallySpacedRectSide\",\"uuid\":\"4b3edad1-18f8-43fa-96ee-a24bb3384b59\"},{\"content\":{\"connectorIds\":[\"In2\"],\"side\":\"TOP\"},\"type\":\"ConnectorPlacement.EquallySpacedRectSide\",\"uuid\":\"43d4f51d-f841-40d6-804e-7f238a90dabe\"},{\"content\":{\"connectorIds\":[\"In3\"],\"side\":\"BOTTOM\"},\"type\":\"ConnectorPlacement.EquallySpacedRectSide\",\"uuid\":\"350f2274-4108-4e6e-a637-0ae7118de3f0\"}]},\"type\":\"ConnectorPlacement.EquallySpacedConnector\",\"uuid\":\"d7e795ea-9d5d-4a8c-83ab-dab42197cc2f\"}],\"packageUris\":[\"http://schema.mathworks.com/mf0/Connector/R2020b\"],\"version\":\"1.0\"}"
  Inlet : PMIOPort  Side=Left
  Outlet : PMIOPort  Port=2  Side=Right
  XeOut : Outport
  GasOut : Outport  Port=2
  wires:
  XenonCalc/1(XeOut) -> XeOut/1
  Add/1 -> Gain/1
  GasCalc/1(GasOut) -> GasOut/1, Add/2
  Gain/1 -> Delay One Step/1
  GasIn/1 -> GasCalc/1(GasIn), Add/1
  Delay One Step/1 -> XenonCalc/3(GasRef), Subsystem/1(GasInRef)
  XeIn/1 -> XenonCalc/1(XeIn)
  PLossFunc/1(PLoss) -> XenonCalc/2(PLoss)
  connections:
  GasCalc/LConn1 -- XenonCalc/LConn1 -- Inlet/RConn1
  GasCalc/LConn3 -- PLossFunc/RConn1 -- Outlet/RConn1 -- Subsystem/RConn1
  GasCalc/LConn2 -- Subsystem/RConn2
  PLossFunc/LConn1 -- XenonCalc/RConn1 -- Subsystem/LConn1

== system MSDRPrimaryLoop_LoadFollow/pipePumpToPHX ==
  XeIn : Inport
  GasIn : Inport  Port=2
  Add : Sum  Inputs=|++
  Delay One Step : Delay  DelayLength=1
  Gain : Gain  Gain=0.5
  GasCalc : Subsystem  mask{Volume=Volume}
      settings: PortSchema="{\"entries\":[{\"content\":{\"sides\":[{\"content\":{\"connectorIds\":[\"In1\"]},\"type\":\"ConnectorPlacement.EquallySpacedRectSide\",\"uuid\":\"a8e1ce06-71c9-462d-8d5c-7a3e078b5544\"},{\"content\":{\"connectorIds\":[\"Out1\"],\"side\":\"RIGHT\"},\"type\":\"ConnectorPlacement.EquallySpacedRectSide\",\"uuid\":\"2c63a1ce-15e2-4b17-a432-f9f40781bd58\"},{\"content\":{\"connectorIds\":[\"LConn1\",\"LConn2\",\"LConn3\"],\"side\":\"TOP\"},\"type\":\"ConnectorPlacement.EquallySpacedRectSide\",\"uuid\":\"abc20e07-15eb-475f-be7f-cc96378523a1\"},{\"content\":{\"connectorIds\":[],\"side\":\"BOTTOM\"},\"type\":\"ConnectorPlacement.EquallySpacedRectSide\",\"uuid\":\"ab58f362-f4c2-4e86-bda0-802426066295\"}]},\"type\":\"ConnectorPlacement.EquallySpacedConnector\",\"uuid\":\"b54d49a9-048b-4912-bf18-92a7ef5e8aff\"}],\"packageUris\":[\"http://schema.mathworks.com/mf0/Connector/R2020b\"],\"version\":\"1.0\"}"
  PLossFunc : Subsystem
      settings: PortSchema="{\"entries\":[{\"content\":{\"sides\":[{\"content\":{\"connectorIds\":[\"Out1\",\"LConn1\"]},\"type\":\"ConnectorPlacement.EquallySpacedRectSide\",\"uuid\":\"95ca4545-c473-4e31-844b-c43557042c16\"},{\"content\":{\"connectorIds\":[\"RConn1\"],\"side\":\"RIGHT\"},\"type\":\"ConnectorPlacement.EquallySpacedRectSide\",\"uuid\":\"f9304c30-8684-4a05-a34b-3121610e628d\"},{\"content\":{\"connectorIds\":[],\"side\":\"TOP\"},\"type\":\"ConnectorPlacement.EquallySpacedRectSide\",\"uuid\":\"64c7a4d8-8539-4303-ae81-4015bd1451af\"}]},\"type\":\"ConnectorPlacement.EquallySpacedConnector\",\"uuid\":\"40c12b2f-fb9d-4a19-b6f1-e93ae1fd4d68\"}],\"packageUris\":[\"http://schema.mathworks.com/mf0/Connector/R2020b\"],\"version\":\"1.0\"}"
  Subsystem : Subsystem  mask{Volume=Volume, Area=Area, Length=Length, Dh=Dh, Elevation=Elevation}
      mask prompts: Dh "Hydraulic Diameter"
      settings: PortSchema="{\"entries\":[{\"content\":{\"sides\":[{\"content\":{\"connectorIds\":[\"LConn1\",\"In1\"]},\"type\":\"ConnectorPlacement.EquallySpacedRectSide\",\"uuid\":\"0f255306-ec83-4423-ac41-a2708bd1ec44\"},{\"content\":{\"connectorIds\":[\"RConn1\"],\"side\":\"RIGHT\"},\"type\":\"ConnectorPlacement.EquallySpacedRectSide\",\"uuid\":\"650fb4ea-7b32-4c45-8538-9785d9ca64bf\"},{\"content\":{\"connectorIds\":[],\"side\":\"TOP\"},\"type\":\"ConnectorPlacement.EquallySpacedRectSide\",\"uuid\":\"434d3568-54a4-4787-a287-69f15ef478cb\"},{\"content\":{\"connectorIds\":[\"RConn2\"],\"side\":\"BOTTOM\"},\"type\":\"ConnectorPlacement.EquallySpacedRectSide\",\"uuid\":\"5b0b510d-1175-4508-bbe9-65b563e28484\"}]},\"type\":\"ConnectorPlacement.EquallySpacedConnector\",\"uuid\":\"b18d9c84-3d71-444b-a89d-79c3dc70d4d9\"}],\"packageUris\":[\"http://schema.mathworks.com/mf0/Connector/R2020b\"],\"version\":\"1.0\"}"
  XenonCalc : Subsystem  mask{Volume=Volume, Area=Area, Length=Length, Dh=Dh, Elevation=Elevation}
      mask prompts: Dh "Hydraulic Diameter"
      settings: PortSchema="{\"entries\":[{\"content\":{\"sides\":[{\"content\":{\"connectorIds\":[\"LConn1\",\"In1\"]},\"type\":\"ConnectorPlacement.EquallySpacedRectSide\",\"uuid\":\"82f8e7e7-fd89-4597-952e-64db268d0190\"},{\"content\":{\"connectorIds\":[\"RConn1\",\"Out1\"],\"side\":\"RIGHT\"},\"type\":\"ConnectorPlacement.EquallySpacedRectSide\",\"uuid\":\"4b3edad1-18f8-43fa-96ee-a24bb3384b59\"},{\"content\":{\"connectorIds\":[\"In2\"],\"side\":\"TOP\"},\"type\":\"ConnectorPlacement.EquallySpacedRectSide\",\"uuid\":\"43d4f51d-f841-40d6-804e-7f238a90dabe\"},{\"content\":{\"connectorIds\":[\"In3\"],\"side\":\"BOTTOM\"},\"type\":\"ConnectorPlacement.EquallySpacedRectSide\",\"uuid\":\"350f2274-4108-4e6e-a637-0ae7118de3f0\"}]},\"type\":\"ConnectorPlacement.EquallySpacedConnector\",\"uuid\":\"d7e795ea-9d5d-4a8c-83ab-dab42197cc2f\"}],\"packageUris\":[\"http://schema.mathworks.com/mf0/Connector/R2020b\"],\"version\":\"1.0\"}"
  Inlet : PMIOPort  Side=Left
  Outlet : PMIOPort  Port=2  Side=Right
  XeOut : Outport
  GasOut : Outport  Port=2
  wires:
  XenonCalc/1(XeOut) -> XeOut/1
  Add/1 -> Gain/1
  GasCalc/1(GasOut) -> GasOut/1, Add/2
  Gain/1 -> Delay One Step/1
  GasIn/1 -> GasCalc/1(GasIn), Add/1
  Delay One Step/1 -> XenonCalc/3(GasRef), Subsystem/1(GasInRef)
  XeIn/1 -> XenonCalc/1(XeIn)
  PLossFunc/1(PLoss) -> XenonCalc/2(PLoss)
  connections:
  GasCalc/LConn1 -- XenonCalc/LConn1 -- Inlet/RConn1
  GasCalc/LConn3 -- PLossFunc/RConn1 -- Outlet/RConn1 -- Subsystem/RConn1
  GasCalc/LConn2 -- Subsystem/RConn2
  PLossFunc/LConn1 -- XenonCalc/RConn1 -- Subsystem/LConn1

== system MSDRPrimaryLoop_LoadFollow/pipeReactorToPump ==
  XeIn : Inport
  GasIn : Inport  Port=2
  Add : Sum  Inputs=|++
  Delay One Step : Delay  DelayLength=1
  Gain : Gain  Gain=0.5
  GasCalc : Subsystem  mask{Volume=Volume}
      settings: PortSchema="{\"entries\":[{\"content\":{\"sides\":[{\"content\":{\"connectorIds\":[\"In1\"]},\"type\":\"ConnectorPlacement.EquallySpacedRectSide\",\"uuid\":\"a8e1ce06-71c9-462d-8d5c-7a3e078b5544\"},{\"content\":{\"connectorIds\":[\"Out1\"],\"side\":\"RIGHT\"},\"type\":\"ConnectorPlacement.EquallySpacedRectSide\",\"uuid\":\"2c63a1ce-15e2-4b17-a432-f9f40781bd58\"},{\"content\":{\"connectorIds\":[\"LConn1\",\"LConn2\",\"LConn3\"],\"side\":\"TOP\"},\"type\":\"ConnectorPlacement.EquallySpacedRectSide\",\"uuid\":\"abc20e07-15eb-475f-be7f-cc96378523a1\"},{\"content\":{\"connectorIds\":[],\"side\":\"BOTTOM\"},\"type\":\"ConnectorPlacement.EquallySpacedRectSide\",\"uuid\":\"ab58f362-f4c2-4e86-bda0-802426066295\"}]},\"type\":\"ConnectorPlacement.EquallySpacedConnector\",\"uuid\":\"b54d49a9-048b-4912-bf18-92a7ef5e8aff\"}],\"packageUris\":[\"http://schema.mathworks.com/mf0/Connector/R2020b\"],\"version\":\"1.0\"}"
  PLossFunc : Subsystem
      settings: PortSchema="{\"entries\":[{\"content\":{\"sides\":[{\"content\":{\"connectorIds\":[\"Out1\",\"LConn1\"]},\"type\":\"ConnectorPlacement.EquallySpacedRectSide\",\"uuid\":\"95ca4545-c473-4e31-844b-c43557042c16\"},{\"content\":{\"connectorIds\":[\"RConn1\"],\"side\":\"RIGHT\"},\"type\":\"ConnectorPlacement.EquallySpacedRectSide\",\"uuid\":\"f9304c30-8684-4a05-a34b-3121610e628d\"},{\"content\":{\"connectorIds\":[],\"side\":\"TOP\"},\"type\":\"ConnectorPlacement.EquallySpacedRectSide\",\"uuid\":\"64c7a4d8-8539-4303-ae81-4015bd1451af\"}]},\"type\":\"ConnectorPlacement.EquallySpacedConnector\",\"uuid\":\"40c12b2f-fb9d-4a19-b6f1-e93ae1fd4d68\"}],\"packageUris\":[\"http://schema.mathworks.com/mf0/Connector/R2020b\"],\"version\":\"1.0\"}"
  Subsystem : Subsystem  mask{Volume=Volume, Area=Area, Length=Length, Dh=Dh, Elevation=Elevation}
      mask prompts: Dh "Hydraulic Diameter"
      settings: PortSchema="{\"entries\":[{\"content\":{\"sides\":[{\"content\":{\"connectorIds\":[\"LConn1\",\"In1\"]},\"type\":\"ConnectorPlacement.EquallySpacedRectSide\",\"uuid\":\"0f255306-ec83-4423-ac41-a2708bd1ec44\"},{\"content\":{\"connectorIds\":[\"RConn1\"],\"side\":\"RIGHT\"},\"type\":\"ConnectorPlacement.EquallySpacedRectSide\",\"uuid\":\"650fb4ea-7b32-4c45-8538-9785d9ca64bf\"},{\"content\":{\"connectorIds\":[],\"side\":\"TOP\"},\"type\":\"ConnectorPlacement.EquallySpacedRectSide\",\"uuid\":\"434d3568-54a4-4787-a287-69f15ef478cb\"},{\"content\":{\"connectorIds\":[\"RConn2\"],\"side\":\"BOTTOM\"},\"type\":\"ConnectorPlacement.EquallySpacedRectSide\",\"uuid\":\"5b0b510d-1175-4508-bbe9-65b563e28484\"}]},\"type\":\"ConnectorPlacement.EquallySpacedConnector\",\"uuid\":\"b18d9c84-3d71-444b-a89d-79c3dc70d4d9\"}],\"packageUris\":[\"http://schema.mathworks.com/mf0/Connector/R2020b\"],\"version\":\"1.0\"}"
  XenonCalc : Subsystem  mask{Volume=Volume, Area=Area, Length=Length, Dh=Dh, Elevation=Elevation}
      mask prompts: Dh "Hydraulic Diameter"
      settings: PortSchema="{\"entries\":[{\"content\":{\"sides\":[{\"content\":{\"connectorIds\":[\"LConn1\",\"In1\"]},\"type\":\"ConnectorPlacement.EquallySpacedRectSide\",\"uuid\":\"82f8e7e7-fd89-4597-952e-64db268d0190\"},{\"content\":{\"connectorIds\":[\"RConn1\",\"Out1\"],\"side\":\"RIGHT\"},\"type\":\"ConnectorPlacement.EquallySpacedRectSide\",\"uuid\":\"4b3edad1-18f8-43fa-96ee-a24bb3384b59\"},{\"content\":{\"connectorIds\":[\"In2\"],\"side\":\"TOP\"},\"type\":\"ConnectorPlacement.EquallySpacedRectSide\",\"uuid\":\"43d4f51d-f841-40d6-804e-7f238a90dabe\"},{\"content\":{\"connectorIds\":[\"In3\"],\"side\":\"BOTTOM\"},\"type\":\"ConnectorPlacement.EquallySpacedRectSide\",\"uuid\":\"350f2274-4108-4e6e-a637-0ae7118de3f0\"}]},\"type\":\"ConnectorPlacement.EquallySpacedConnector\",\"uuid\":\"d7e795ea-9d5d-4a8c-83ab-dab42197cc2f\"}],\"packageUris\":[\"http://schema.mathworks.com/mf0/Connector/R2020b\"],\"version\":\"1.0\"}"
  Inlet : PMIOPort  Side=Left
  Outlet : PMIOPort  Port=2  Side=Right
  XeOut : Outport
  GasOut : Outport  Port=2
  wires:
  XenonCalc/1(XeOut) -> XeOut/1
  Add/1 -> Gain/1
  GasCalc/1(GasOut) -> GasOut/1, Add/2
  Gain/1 -> Delay One Step/1
  GasIn/1 -> GasCalc/1(GasIn), Add/1
  Delay One Step/1 -> XenonCalc/3(GasRef), Subsystem/1(GasInRef)
  XeIn/1 -> XenonCalc/1(XeIn)
  PLossFunc/1(PLoss) -> XenonCalc/2(PLoss)
  connections:
  GasCalc/LConn1 -- XenonCalc/LConn1 -- Inlet/RConn1
  GasCalc/LConn3 -- PLossFunc/RConn1 -- Outlet/RConn1 -- Subsystem/RConn1
  GasCalc/LConn2 -- Subsystem/RConn2
  PLossFunc/LConn1 -- XenonCalc/RConn1 -- Subsystem/LConn1
